simulink model "sl_subsys_swerr1"  (Simulink 7.6)
settings: Solver=FixedStepDiscrete  StartTime=0.0  StopTime=10.0  FixedStep=1  RelTol=1e-3
Description:
  | Switch-case block and action subsystem illegal example
  | 
  | This following model is an example of an illegal  combination of a switch-case block executing
  | the action subsystem 'case body'. Block B is driving the 'case body' block and
  | must execute before the 'Switch-case' block. However, the 'case body' block needs to execute
  | before 'B'. This poses a causality problem.  To execute 'case body', we must
  | first execute 'Switch-case', before 'B'. However, 'B' must execute prior to
  | "Switch-case' and, hence, the error.
settings Model: Creator=The MathWorks Inc.  CovMetricSettings=d  ExtModeAutoUpdateStatusClock=off
settings OptimizationCC: BlockReduction=off  BooleanDataType=off  InlineInvariantSignals=on  InitFltsAndDblsToZero=on
settings DebuggingCC: SaveWithParameterizedLinksMsg=none  SignalResolutionControl=TryResolveAllWithWarning  SolverPrmCheckMsg=none  MultiTaskDSMMsg=warning  MultiTaskCondExecSysMsg=none
settings HardwareCC: TargetUnknown=on
settings RTWCC: IncludeERTFirstTime=on
settings CodeAppCC: CustomSymbolStrFcn=$F$N$M
settings GRTTargetCC: TargetFcnLib=ansi_tfl_tmw.mat

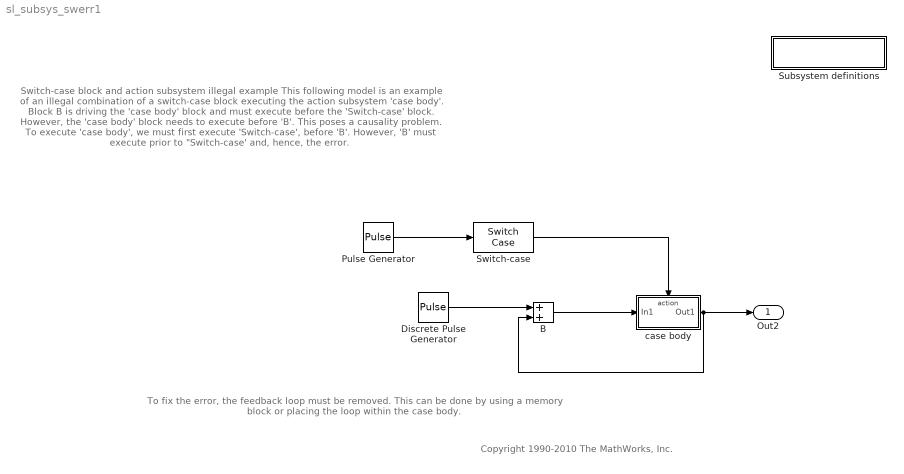
== system sl_subsys_swerr1 ==
  note: To fix the error, the feedback loop must be removed. This can be done by
      | using a memory block or placing the loop within the case body.
  note: Switch-case block and action subsystem illegal example
      |
      | This following model is an example of an illegal  combination of a switch-case block executing
      | the action subsystem 'case body'. Block B is driving the 'case body' block and
      | must execute before the 'Switch-case' block. However, the 'case body' block needs to execute
      | before 'B'. This poses a causality problem.  To execute 'case body', we must
      | first execute 'Switch-case', before 'B'. However, 'B' must execute prior to
      | "Switch-case' and, hence, the error.
  note: Copyright 1990-2010 The MathWorks, Inc.
  " Subsystem definitions" : Subsystem
      settings: OpenFcn=helpview([matlabroot,'/toolbox/simulink/simdemos/simfeatures/html/sl_subsys_definitions.html']);
      mask Display: disp('Subsystem\ndefinitions')
  B : Sum  SaturateOnIntegerOverflow=on  InputSameDT=on  OutDataTypeStr=Inherit: Same as first input
  Discrete Pulse Generator : DiscretePulseGenerator
  Pulse Generator : DiscretePulseGenerator
  Switch-case : SwitchCase  ShowDefaultCase=off
  case body : Subsystem  TreatAsAtomicUnit=on
  Out2 : Outport
  wires:
  Switch-case/1 -> case body/Action
  B/1 -> case body/1(In1)
  Pulse Generator/1 -> Switch-case/1
  Discrete Pulse Generator/1 -> B/1
  case body/1(Out1) -> B/2, Out2/1

== system sl_subsys_swerr1/ Subsystem definitions ==

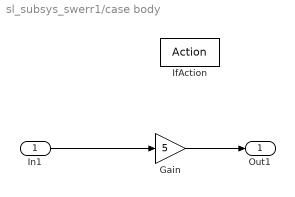
== system sl_subsys_swerr1/case body ==
  In1 : Inport
  IfAction : ActionPort  ActionType=case
  Gain : Gain  Gain=5  SaturateOnIntegerOverflow=on  OutDataTypeStr=Inherit: Same as input  ParamDataTypeStr=Inherit: Same as input
  Out1 : Outport
  wires:
  In1/1 -> Gain/1
  Gain/1 -> Out1/1
